simulink model "Controller0"  (R2020a)
settings: Solver=VariableStepAuto  StartTime=0.0  StopTime=10.0  RelTol=1e-3
values from neighbouring files (symbols this model uses):
  Ts = 0.01    [PID_handon.m]
undefined symbols (not defined in the file or in its folder): Ki, Kp
settings Model: Creator=pawankumarf  LastModifiedBy=Ganesh
settings DataIOCC: ExternalInput=[t, stin]  LoadExternalInput=on  SaveFormat=Array  SaveOutput=off  SaveTime=off  ReturnWorkspaceOutputs=off

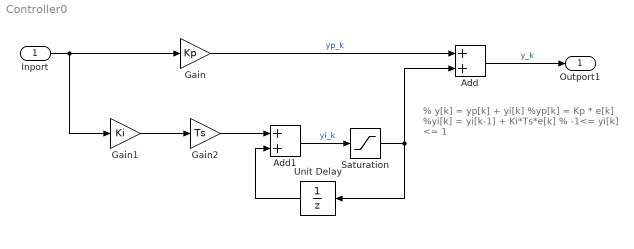
== system Controller0 ==
  note: % y[k] = yp[k] + yi[k]
      | %yp[k] = Kp * e[k]
      | %yi[k] = yi[k-1] + Ki*Ts*e[k]
      | % -1<= yi[k] <= 1
  Inport : Inport  OutDataTypeStr=double  PortDimensions=1  SampleTime=0
  Add : Sum
  Add1 : Sum
  Gain : Gain  Gain=Kp
  Gain1 : Gain  Gain=Ki
  Gain2 : Gain  Gain=Ts
  Saturation : Saturate  UpperLimit=1  LowerLimit=-1
  Unit Delay : UnitDelay  SampleTime=-1  HasFrameUpgradeWarning=on
  Outport1 : Outport  OutDataTypeStr=double  PortDimensions=1  SampleTime=0
  wires:
  Gain/1 -> Add/1  "yp_k"
  Gain2/1 -> Add1/1
  Add/1 -> Outport1/1  "y_k"
  Inport/1 -> Gain/1, Gain1/1
  Gain1/1 -> Gain2/1
  Unit Delay/1 -> Add1/2
  Saturation/1 -> Unit Delay/1, Add/2
  Add1/1 -> Saturation/1  "yi_k"
